simulink model "Inverted_Spring_pendulum_on_a_cart_SIMULINK"  (R2023b)
settings: Solver=FixedStepAuto  StartTime=0.0  StopTime=30  FixedStep=0.1  RelTol=1e-3
settings Model: Creator=Bhawn  LastModifiedBy=Bhawn

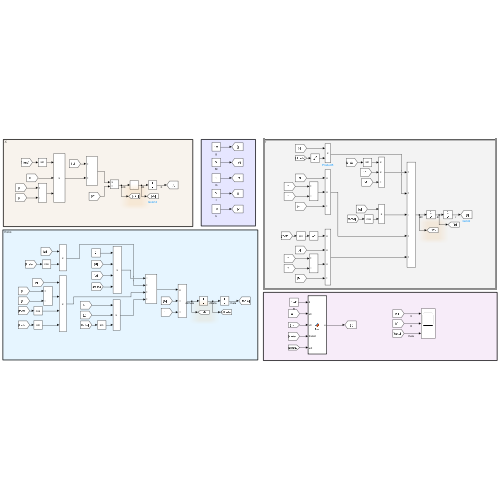
[thumbnail: Simulink's stored preview of the top-level diagram]
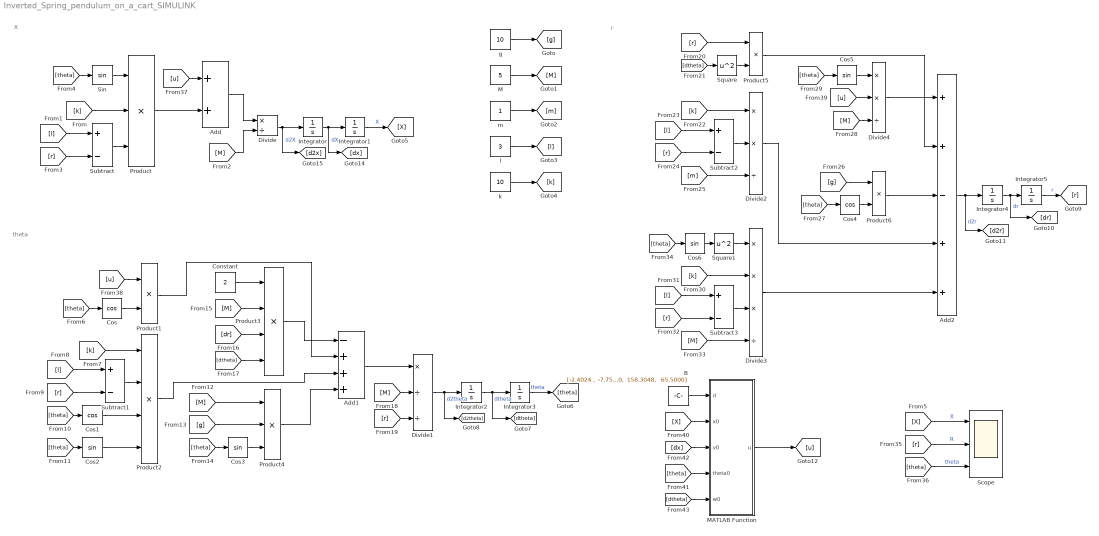
== system Inverted_Spring_pendulum_on_a_cart_SIMULINK ==
  note: r
  note: theta
  note: X
  Add : Sum
  Add1 : Sum  Inputs=-+++
  Add2 : Sum  Inputs=++-++
  B : Constant  Value="[-2.4024 ,  -7.7500,  158.3048,   65.5000]"
  Constant : Constant  Value=2
  Cos : Trigonometry  Operator=cos
  Cos1 : Trigonometry  Operator=cos
  Cos{2..3,5..6} (4 alike) : Trigonometry
  Cos4 : Trigonometry  Operator=cos
  Divide : Product  Inputs=*/
  Divide1 : Product  Inputs=*//
  Divide2 : Product  Inputs=**/
  Divide3 : Product  Inputs=***/
  Divide4 : Product  Inputs=**/
  Integrator{,1..2,4} (4 alike) : Integrator
  Integrator3 : Integrator  InitialCondition=0.1
  Integrator5 : Integrator  InitialCondition=2
  M : Constant  Value=5
  MATLAB Function : MATLAB Function  TreatAsAtomicUnit=on
  Product : Product  Inputs=3
  Product1 : Product
  Product2 : Product  Inputs=4
  Product3 : Product  Inputs=4
  Product4 : Product  Inputs=3
  Product5 : Product
  Product6 : Product
  Scope : Scope  NumInputPorts=3
  Sin : Trigonometry
  Square : Math  Operator=square
  Square1 : Math  Operator=square
  Subtract{,1..3} (4 alike) : Sum  Inputs=+-
  g : Constant  Value=10
  k : Constant  Value=10
  l : Constant  Value=3
  m : Constant
  wires:
  m/1 -> [m]
  k/1 -> [k]
  l/1 -> [l]
  g/1 -> [g]
  M/1 -> [M]
  [l] -> Subtract/1
  [r] -> Subtract/2
  [theta] -> Sin/1
  Sin/1 -> Product/1
  [k] -> Product/2
  Subtract/1 -> Product/3
  Add/1 -> Divide/1
  [M] -> Divide/2
  Divide/1 -> [d2x], Integrator/1  "d2X"
  Integrator/1 -> [dx], Integrator1/1  "dX"
  Integrator1/1 -> [X]  "X"
  [u] -> Add/1
  Product/1 -> Add/2
  [theta] -> Cos/1
  [u] -> Product1/1
  Cos/1 -> Product1/2
  [r] -> Subtract1/2
  [k] -> Product2/1
  [l] -> Subtract1/1
  Subtract1/1 -> Product2/2
  [theta] -> Cos2/1
  [theta] -> Cos1/1
  Cos1/1 -> Product2/3
  Cos2/1 -> Product2/4
  [theta] -> Cos3/1
  Constant/1 -> Product3/1
  [M] -> Product3/2
  [dr] -> Product3/3
  [dtheta] -> Product3/4
  [M] -> Product4/1
  [g] -> Product4/2
  Cos3/1 -> Product4/3
  Product3/1 -> Add1/1
  Product4/1 -> Add1/4
  Product2/1 -> Add1/3
  Product1/1 -> Add1/2
  Add1/1 -> Divide1/1
  [M] -> Divide1/2
  [r] -> Divide1/3
  Divide1/1 -> [d2theta], Integrator2/1  "d2theta"
  Integrator2/1 -> [dtheta], Integrator3/1  "dtheta"
  Integrator3/1 -> [theta]  "theta"
  [dtheta] -> Square/1
  [l] -> Subtract2/1
  [k] -> Divide2/1
  [r] -> Subtract2/2
  Subtract2/1 -> Divide2/2
  [m] -> Divide2/3
  [theta] -> Cos4/1
  Subtract3/1 -> Divide3/3
  [M] -> Divide3/4
  [l] -> Subtract3/1
  [r] -> Subtract3/2
  [k] -> Divide3/2
  [theta] -> Cos6/1
  Cos6/1 -> Square1/1
  Square1/1 -> Divide3/1
  [r] -> Product5/1
  Square/1 -> Product5/2
  Cos4/1 -> Product6/2
  [g] -> Product6/1
  [theta] -> Cos5/1
  Cos5/1 -> Divide4/1
  [u] -> Divide4/2
  [M] -> Divide4/3
  Divide4/1 -> Add2/1
  Product5/1 -> Add2/2
  Divide3/1 -> Add2/5
  Divide2/1 -> Add2/4
  Product6/1 -> Add2/3
  Add2/1 -> [d2r], Integrator4/1  "d2r"
  Integrator4/1 -> [dr], Integrator5/1  "dr"
  Integrator5/1 -> [r]  "r"
  [X] -> Scope/1  "X"
  [r] -> Scope/2  "R"
  [theta] -> Scope/3  "theta"
  B/1 -> MATLAB Function/1(d)
  [X] -> MATLAB Function/2(x0)
  [theta] -> MATLAB Function/4(theta0)
  MATLAB Function/1(u) -> [u]
  [dtheta] -> MATLAB Function/5(w0)
  [dx] -> MATLAB Function/3(v0)

== matlab function Inverted_Spring_pendulum_on_a_cart_SIMULINK/MATLAB Function ==
  data: u output; d input; x0 input; v0 input; theta0 input; w0 input
function u = fcn(d, x0, v0, theta0,w0)
X=[x0-0; v0-0; theta0-0; w0-0];
p=dot(d,X);
u=-p;
end
